simulink model "Ex3_Antenna_Array_Integration_GECK"  (R2025b)
settings: Solver=VariableStepAuto  StartTime=0.0  StopTime=0.01  RelTol=1e-3
InitFcn:
  | fs     = 1e6;
  | Ts     = 1/fs;
  | fc     = 2.4e9;
  | c      = physconst('Lightspeed');
  | lambda = freq2wavelen(fc,c);
libraries: dspstat3 x4, phasedtxrxlib x1
settings Model: Creator=galberti  LastModifiedBy=galberti

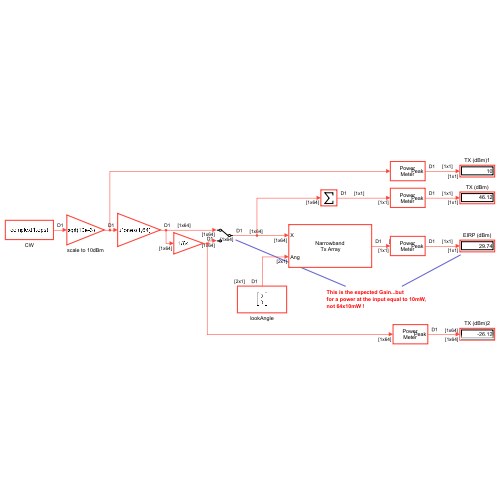
[thumbnail: Simulink's stored preview of the top-level diagram]
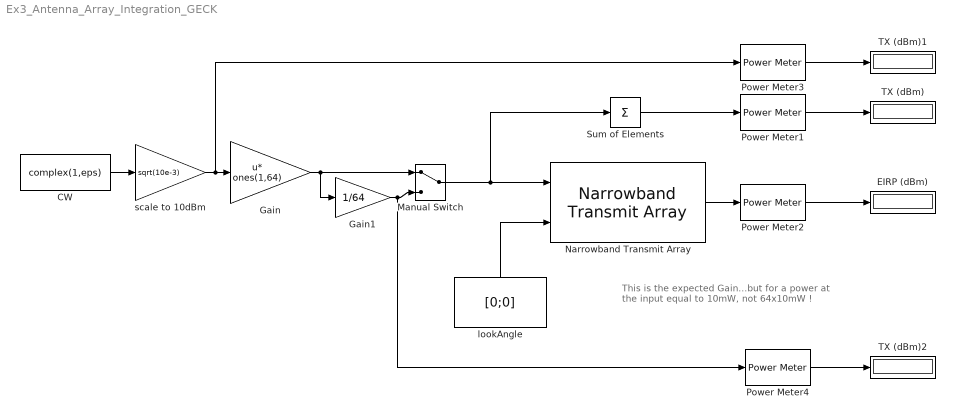
== system Ex3_Antenna_Array_Integration_GECK ==
  note: This is the expected Gain...but
      | for a power at the input equal to 10mW,
      | not 64x10mW !
  CW : Constant  Value=complex(1,eps)  SampleTime=Ts
  EIRP (dBm) : Display
  Gain : Gain  Gain=ones(1,64)  Multiplication=Matrix(u*K)
  Gain1 : Gain  Gain=1/64
  Manual Switch : ManualSwitch
  Narrowband Transmit Array : phasedtxrxlib/Narrowband Transmit Array  PropagationSpeed=c  OperatingFrequency=fc  CombineRadiatedSignals=on  SensorGainMeasure=dBi  Polarization=None  WeightsInputPort=off  SimulateUsing=Interpreted execution  Sensor=phased.URA(Size=[8,8],ElementSpacing=[ 0.5, 0.5 ] .*lambda,ArrayNormal='x',Element=phased.IsotropicAntennaElement())
  Power Meter{1..4} (4 alike) : dspstat3/Power Meter  Measurement=Peak power  ReferenceLoad=1  OutputPowerUnits=dBm  WindowLength=256  OverlapLength=255  AllowArbitraryInputLength=off  ComputeCCDF=off  PowerRange=50  PowerResolution=0.1  CCDFOutput=Relative power (dB above average power)  ProbabilityVector=[ 10; 1; 0.1; 0.01; 0.001; 0.0001 ]  RelativePowerVector=[ 0; 3; 6; 9; 12 ]  ResetPort=off  SimulateUsing=Interpreted execution
      settings: LibrarySourceBlock=commutil2/Power Meter
  Sum of Elements : Sum  Inputs=+  CollapseMode=Specified dimension  CollapseDim=2
  TX (dBm) : Display
  TX (dBm)1 : Display
  TX (dBm)2 : Display
  lookAngle : Constant  Value=[0;0]  VectorParams1D=off  SampleTime=Ts
  scale to 10dBm : Gain  Gain=sqrt(10e-3)
  wires:
  lookAngle/1 -> Narrowband Transmit Array/2
  Narrowband Transmit Array/1 -> Power Meter2/1
  Sum of Elements/1 -> Power Meter1/1
  Power Meter1/1 -> TX (dBm)/1
  Power Meter2/1 -> EIRP (dBm)/1
  CW/1 -> scale to 10dBm/1
  scale to 10dBm/1 -> Power Meter3/1, Gain/1
  Power Meter3/1 -> TX (dBm)1/1
  Gain/1 -> Manual Switch/1, Gain1/1
  Manual Switch/1 -> Sum of Elements/1, Narrowband Transmit Array/1
  Gain1/1 -> Power Meter4/1, Manual Switch/2
  Power Meter4/1 -> TX (dBm)2/1
